simulink model "Modeling_of_system"  (R2023b)
settings: Solver=VariableStepAuto  StartTime=0.0  StopTime=10.0  RelTol=1e-3
values from neighbouring files (symbols this model uses):
  Ip = 2    [data_PMSM.m]
  LS = 0.01    [data_PMSM.m]
  R = 1    [data_PMSM.m]
  Vp = 12    [data_PMSM.m]
  W = 300    [data_PMSM.m]
settings Model: Creator=Beshary  LastModifiedBy=Beshary

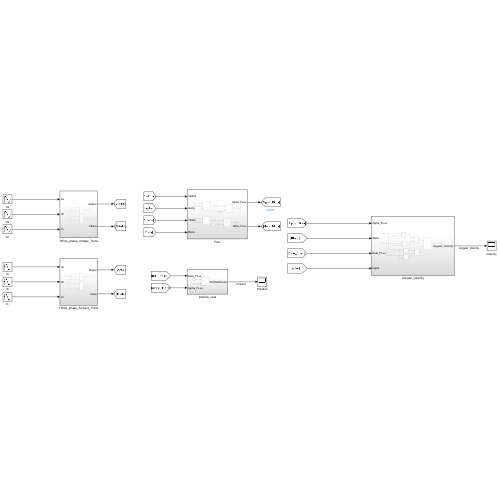
[thumbnail: Simulink's stored preview of the top-level diagram]
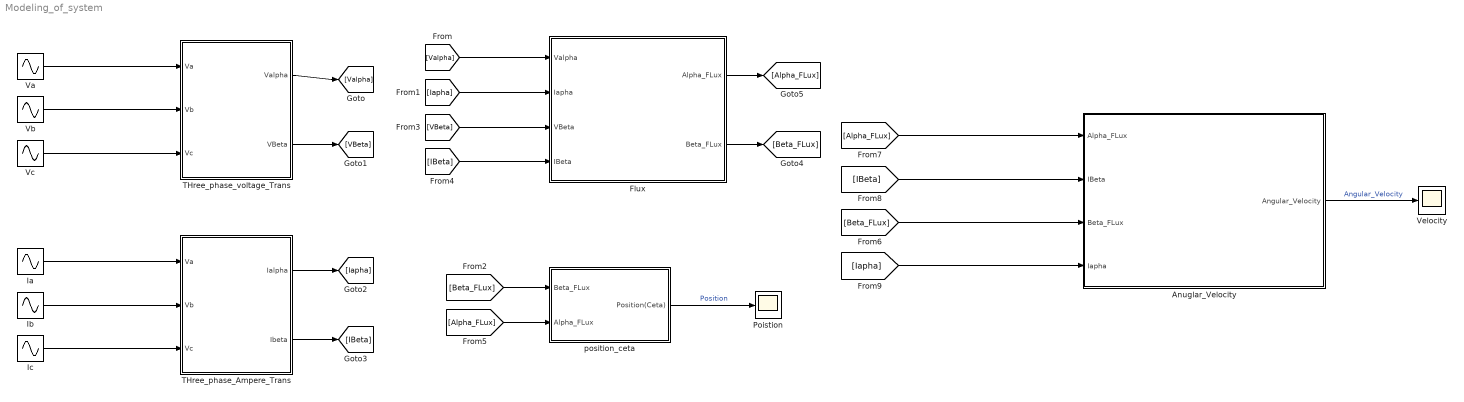
== system Modeling_of_system ==
  Anuglar_Velocity : Subsystem
  Flux : Subsystem
  Ia : Sin  Amplitude=Ip  Frequency=W  SampleTime=0
  Ib : Sin  Amplitude=Ip  Frequency=W  Phase=2*pi/3  SampleTime=0
  Ic : Sin  Amplitude=Ip  Frequency=W  Phase=-2*pi/3  SampleTime=0
  Poistion : Scope
  THree_phase_Ampere_Trans : Subsystem
  THree_phase_voltage_Trans : Subsystem
  Va : Sin  Amplitude=Vp  Frequency=W  SampleTime=0
  Vb : Sin  Amplitude=Vp  Frequency=W  Phase=2*pi/3  SampleTime=0
  Vc : Sin  Amplitude=Vp  Frequency=W  Phase=-2*pi/3  SampleTime=0
  Velocity : Scope
  position_ceta : Subsystem
  wires:
  Va/1 -> THree_phase_voltage_Trans/1(Va)
  Vb/1 -> THree_phase_voltage_Trans/2(Vb)
  Vc/1 -> THree_phase_voltage_Trans/3(Vc)
  Ic/1 -> THree_phase_Ampere_Trans/3(Vc)
  Ib/1 -> THree_phase_Ampere_Trans/2(Vb)
  Ia/1 -> THree_phase_Ampere_Trans/1(Va)
  THree_phase_voltage_Trans/1(Valpha) -> [Valpha]
  THree_phase_voltage_Trans/2(VBeta) -> [VBeta]
  THree_phase_Ampere_Trans/1(Ialpha) -> [Iapha]
  THree_phase_Ampere_Trans/2(Ibeta) -> [IBeta]
  [Valpha] -> Flux/1(Valpha)
  [Iapha] -> Flux/2(Iapha)
  [VBeta] -> Flux/3(VBeta)
  [IBeta] -> Flux/4(IBeta)
  Flux/2(Beta_FLux) -> [Beta_FLux]
  Flux/1(Alpha_FLux) -> [Alpha_FLux]
  [Beta_FLux] -> position_ceta/1(Beta_FLux)
  [Alpha_FLux] -> position_ceta/2(Alpha_FLux)
  position_ceta/1(Position(Ceta)) -> Poistion/1  "Position"
  [Alpha_FLux] -> Anuglar_Velocity/1(Alpha_FLux)
  [IBeta] -> Anuglar_Velocity/2(IBeta)
  [Beta_FLux] -> Anuglar_Velocity/3(Beta_FLux)
  [Iapha] -> Anuglar_Velocity/4(Iapha)
  Anuglar_Velocity/1(Angular_Velocity) -> Velocity/1  "Angular_Velocity"

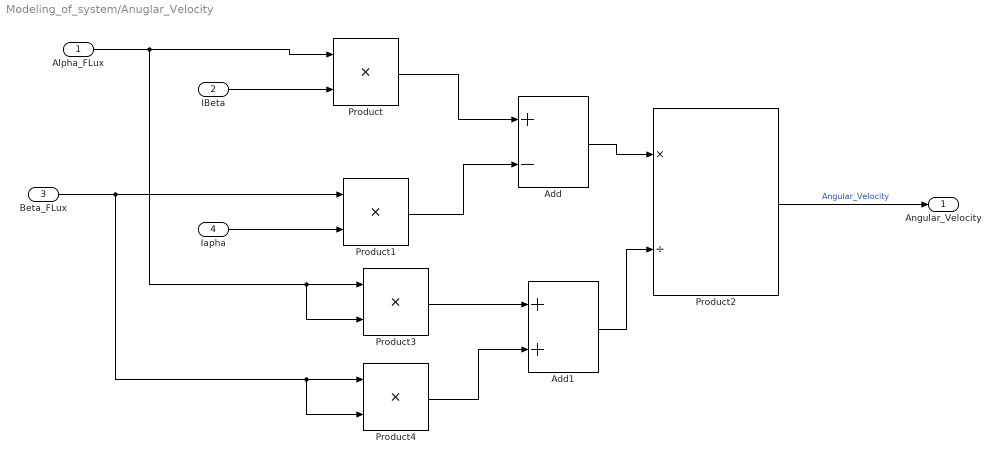
== system Modeling_of_system/Anuglar_Velocity ==
  Alpha_FLux : Inport
  IBeta : Inport  Port=2
  Beta_FLux : Inport  Port=3
  Iapha : Inport  Port=4
  Add : Sum  Inputs=+-
  Add1 : Sum
  Product{,1,3..4} (4 alike) : Product
  Product2 : Product  Inputs=*/
  Angular_Velocity : Outport
  wires:
  IBeta/1 -> Product/2
  Add/1 -> Product2/1
  Product3/1 -> Add1/1
  Beta_FLux/1 -> Product4/1, Product4/2, Product1/1
  Product4/1 -> Add1/2
  Product/1 -> Add/1
  Product1/1 -> Add/2
  Add1/1 -> Product2/2
  Alpha_FLux/1 -> Product/1, Product3/2, Product3/1
  Product2/1 -> Angular_Velocity/1  "Angular_Velocity"
  Iapha/1 -> Product1/2

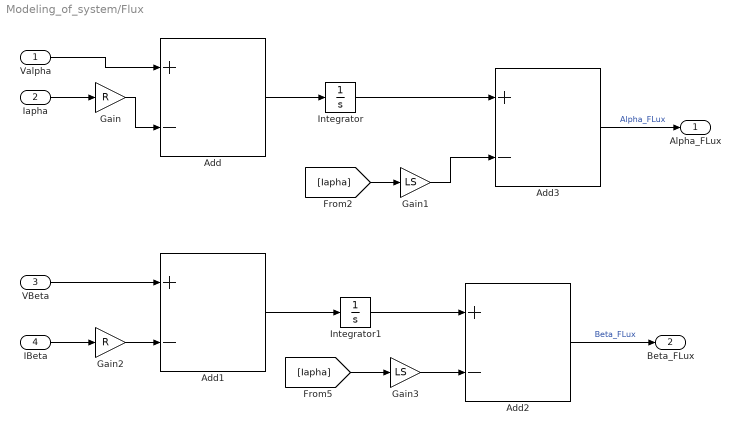
== system Modeling_of_system/Flux ==
  Valpha : Inport
  Iapha : Inport  Port=2
  VBeta : Inport  Port=3
  IBeta : Inport  Port=4
  Add{,1..3} (4 alike) : Sum  Inputs=+-
  Gain : Gain  Gain=R
  Gain1 : Gain  Gain=LS
  Gain2 : Gain  Gain=R
  Gain3 : Gain  Gain=LS
  Integrator : Integrator
  Integrator1 : Integrator
  Alpha_FLux : Outport
  Beta_FLux : Outport  Port=2
  wires:
  [Iapha] -> Gain3/1
  Add1/1 -> Integrator1/1
  Gain1/1 -> Add3/2
  [Iapha] -> Gain1/1
  Integrator/1 -> Add3/1
  Gain2/1 -> Add1/2
  Integrator1/1 -> Add2/1
  Gain3/1 -> Add2/2
  Gain/1 -> Add/2
  Add/1 -> Integrator/1
  Add3/1 -> Alpha_FLux/1  "Alpha_FLux"
  Valpha/1 -> Add/1
  VBeta/1 -> Add1/1
  IBeta/1 -> Gain2/1
  Add2/1 -> Beta_FLux/1  "Beta_FLux"
  Iapha/1 -> Gain/1

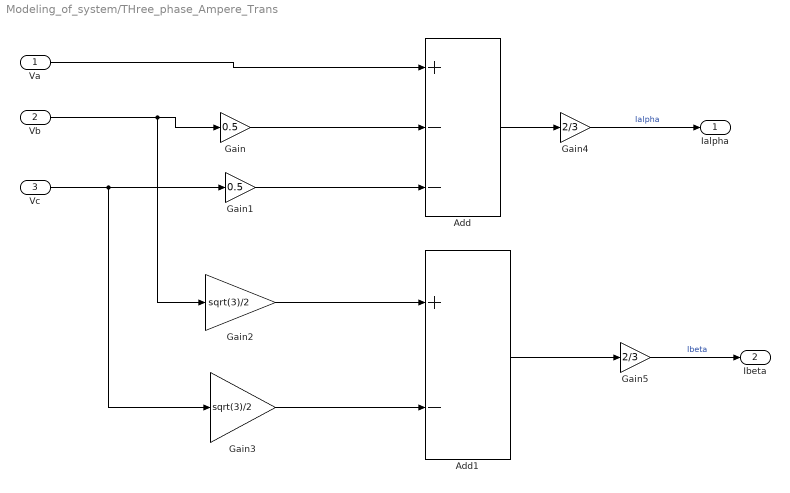
== system Modeling_of_system/THree_phase_Ampere_Trans ==
  Va : Inport
  Vb : Inport  Port=2
  Vc : Inport  Port=3
  Add : Sum  Inputs=+--
  Add1 : Sum  Inputs=+-
  Gain : Gain  Gain=0.5
  Gain1 : Gain  Gain=0.5
  Gain2 : Gain  Gain=sqrt(3)/2
  Gain3 : Gain  Gain=sqrt(3)/2
  Gain4 : Gain  Gain=2/3
  Gain5 : Gain  Gain=2/3
  Ialpha : Outport
  Ibeta : Outport  Port=2
  wires:
  Gain5/1 -> Ibeta/1  "Ibeta"
  Gain4/1 -> Ialpha/1  "Ialpha"
  Va/1 -> Add/1
  Gain2/1 -> Add1/1
  Add1/1 -> Gain5/1
  Gain/1 -> Add/2
  Gain1/1 -> Add/3
  Vc/1 -> Gain1/1, Gain3/1
  Vb/1 -> Gain/1, Gain2/1
  Add/1 -> Gain4/1
  Gain3/1 -> Add1/2

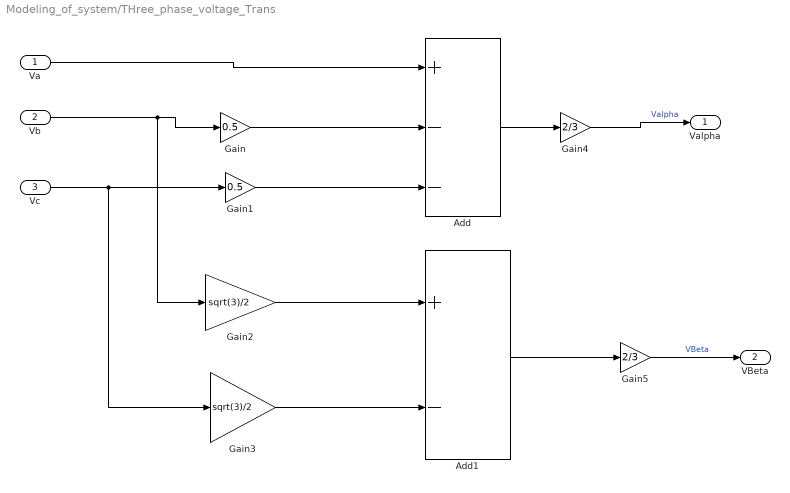
== system Modeling_of_system/THree_phase_voltage_Trans ==
  Va : Inport
  Vb : Inport  Port=2
  Vc : Inport  Port=3
  Add : Sum  Inputs=+--
  Add1 : Sum  Inputs=+-
  Gain : Gain  Gain=0.5
  Gain1 : Gain  Gain=0.5
  Gain2 : Gain  Gain=sqrt(3)/2
  Gain3 : Gain  Gain=sqrt(3)/2
  Gain4 : Gain  Gain=2/3
  Gain5 : Gain  Gain=2/3
  Valpha : Outport
  VBeta : Outport  Port=2
  wires:
  Gain3/1 -> Add1/2
  Add/1 -> Gain4/1
  Vb/1 -> Gain2/1, Gain/1
  Vc/1 -> Gain3/1, Gain1/1
  Gain1/1 -> Add/3
  Gain/1 -> Add/2
  Add1/1 -> Gain5/1
  Gain2/1 -> Add1/1
  Va/1 -> Add/1
  Gain4/1 -> Valpha/1  "Valpha"
  Gain5/1 -> VBeta/1  "VBeta"

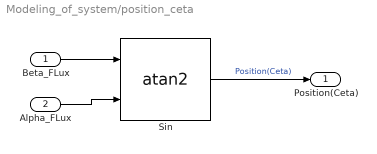
== system Modeling_of_system/position_ceta ==
  Beta_FLux : Inport
  Alpha_FLux : Inport  Port=2
  Sin : Trigonometry  Operator=atan2
  Position(Ceta) : Outport
  wires:
  Beta_FLux/1 -> Sin/1
  Alpha_FLux/1 -> Sin/2
  Sin/1 -> Position(Ceta)/1  "Position(Ceta)"
